simulink model "DrivePurePursuitSquat"  (R2025b)
settings: Solver=VariableStepAuto  StartTime=0.0  StopTime=120  RelTol=0.01  AbsTol=0.01  EnableMultiTasking=on
undefined symbols (not defined in the file): waypoints, X, Y, Z
libraries: sm_lib x71, nesl_utility x45, slpidlib x2, robotalgslib x1, sharedtransform x1
(part 4 of 4)

== system DrivePurePursuitSquat/Subsystem5 ==
  In2 : Inport
  wR_cmd : Inport  Port=2
  PID Controller : slpidlib/PID Controller  Controller=PID  Form=Parallel  TimeDomain=Continuous-time  UseExternalTs=off  SampleTime=-1  IntegratorMethod=Forward Euler  FilterMethod=Forward Euler  ControllerParametersSource=internal  P=5  I=0  UseKiTs=off  D=0  UseExternalDerivativeSource=off  N=100  UseFilter=on  TunerSelectOption=Transfer Function Based (PID Tuner App)  InitialConditionSource=internal  InitialConditionForIntegrator=0  InitialConditionForFilter=0  DifferentiatorICPrevScaledInput=0  ExternalReset=none  TrackingMode=off  Kt=1  LimitOutput=off  SatLimitsSource=internal  UpperSaturationLimit=inf  LowerSaturationLimit=-inf  LinearizeAsGain=on  AntiWindupMode=none  Kb=1  LimitIntegrator=off  UpperIntegratorSaturationLimit=inf  LowerIntegratorSaturationLimit=-inf  POutMin=[]  POutMax=[]  IOutMin=[]  IOutMax=[]  DOutMin=[]  DOutMax=[]  NOutMin=[]  NOutMax=[]  SumOutMin=[]  SumOutMax=[]  SaturationOutMin=[]  SaturationOutMax=[]  PParamMin=[]  PParamMax=[]  IParamMin=[]  IParamMax=[]  DParamMin=[]  DParamMax=[]  NParamMin=[]  NParamMax=[]  KbParamMin=[]  KbParamMax=[]  KtParamMin=[]  KtParamMax=[]  KbOutMin=[]  KbOutMax=[]  KtOutMin=[]  KtOutMax=[]  IntegratorOutMin=[]  IntegratorOutMax=[]  FilterOutMin=[]  FilterOutMax=[]  SumI1OutMin=[]  SumI1OutMax=[]  SumI2OutMin=[]  SumI2OutMax=[]  SumI3OutMin=[]  SumI3OutMax=[]  SumI4OutMin=[]  SumI4OutMax=[]  SumDOutMin=[]  SumDOutMax=[]  DifferentiatorOutMin=[]  DifferentiatorOutMax=[]  FilterDiffOutCoefMin=[]  FilterDiffOutCoefMax=[]  ReciprocalOutMin=[]  ReciprocalOutMax=[]  SumDenOutMin=[]  SumDenOutMax=[]  SumNumOutMin=[]  SumNumOutMax=[]  DivideOutMin=[]  DivideOutMax=[]  UdiffTsProdOutMin=[]  UdiffTsProdOutMax=[]  NTsProdOutMin=[]  NTsProdOutMax=[]  UintegralTsProdOutMin=[]  UintegralTsProdOutMax=[]  UngainTsProdOutMin=[]  UngainTsProdOutMax=[]  ClampingZeroOutDataTypeStr=Inherit: Inherit via back propagation  ClampingZeroOutMin=[]  ClampingZeroOutMax=[]  FilterDenConstantOutDataTypeStr=Inherit: Inherit via back propagation  FilterDenConstantOutMin=[]  FilterDenConstantOutMax=[]  PCopyOutDataTypeStr=Inherit: Inherit via back propagation  PCopyOutMin=[]  PCopyOutMax=[]  NCopyOutDataTypeStr=Inherit: Inherit via back propagation  NCopyOutMin=[]  NCopyOutMax=[]  IntegratorContinuousStateAttributes=''  IntegratorStateMustResolveToSignalObject=off  IntegratorRTWStateStorageClass=Auto  FilterContinuousStateAttributes=''  FilterStateMustResolveToSignalObject=off  FilterRTWStateStorageClass=Auto  ParallelPVariant=InternalParameters  IdealPVariant=Disabled  IVariant=InternalParameters  DVariant=InternalParameters  IntegratorVariant=Continuous  SatVariant=Disabled  AWVariant=Passthrough  PCopyVariant=Disabled  TRVariant=Disabled  FdbkBlocksVariant=Forward  IdealPFdbkVariant=Disabled  SatFdbkVariant=Disabled  DerivativeFilterVariant=ContFilter  NVariant=InternalParameters  NCopyVariant=Disabled  FilterICVariant=InternalICsFilter  IntegratorICVariant=InternalICs  ExternalResetVariant=Disabled  TRSumVariant=Passthrough  SumFdbkVariant=Disabled  SumVariant=Sum_PID  TsampFilterVariant=InternalTs  TsampNgainVariant=Passthrough  TsampIntegralVariant=Disabled_SignalSpec  ExternalSaturationOutDataTypeStr=Inherit: Same as second input  DerivativeSourceVariant=ErrorSignal  PreIntVariant=InternalPreInt
  Saturation : Saturate  UpperLimit=5  LowerLimit=-5
  Subtract : Sum  Inputs=+-
  Out1 : Outport
  wires:
  In2/1 -> Subtract/2
  Subtract/1 -> PID Controller/1
  Saturation/1 -> Out1/1
  PID Controller/1 -> Saturation/1
  wR_cmd/1 -> Subtract/1

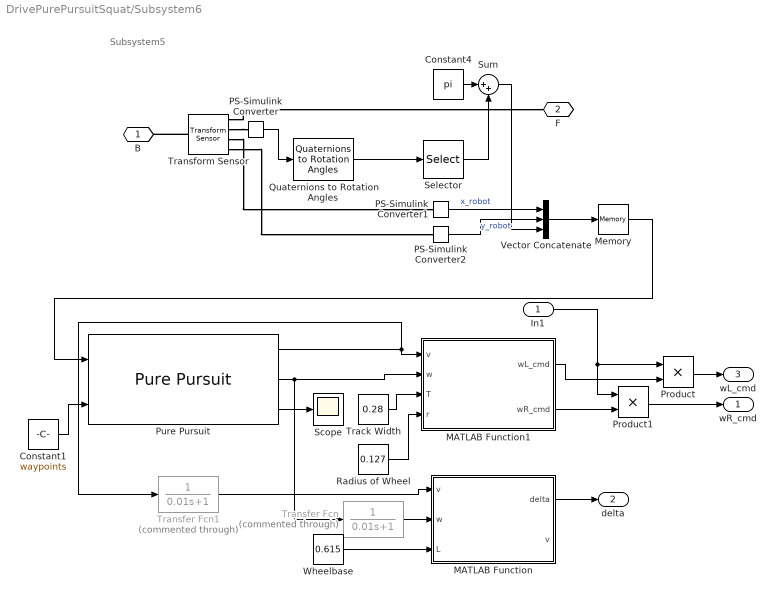
== system DrivePurePursuitSquat/Subsystem6 ==
  note: Subsystem5
  In1 : Inport
  Constant1 : Constant  Value=waypoints
  Constant4 : Constant  Value=pi
  MATLAB Function : MATLAB Function  TreatAsAtomicUnit=on
  MATLAB Function1 : MATLAB Function  TreatAsAtomicUnit=on
  Memory : Memory
  PS-Simulink Converter : nesl_utility/PS-Simulink Converter  PhysicalDomain=network_engine_domain  SubClassName=ps_output  LeftPortType=input  RightPortType=output  PseudoPeriodic=off  Frequencies=[]  VectorFormat=inherit  Unit=inherit  AffineConversion=off
  PS-Simulink Converter1 : nesl_utility/PS-Simulink Converter  PhysicalDomain=network_engine_domain  SubClassName=ps_output  LeftPortType=input  RightPortType=output  PseudoPeriodic=off  Frequencies=[]  VectorFormat=inherit  Unit=inherit  AffineConversion=off
  PS-Simulink Converter2 : nesl_utility/PS-Simulink Converter  PhysicalDomain=network_engine_domain  SubClassName=ps_output  LeftPortType=input  RightPortType=output  PseudoPeriodic=off  Frequencies=[]  VectorFormat=inherit  Unit=inherit  AffineConversion=off
  Product : Product
  Product1 : Product
  Pure Pursuit : robotalgslib/Pure Pursuit  DesiredLinearVelocityPort=off  DesiredLinearVelocity=0.7  MaxAngularVelocity=0.8  LookaheadDistancePort=off  LookaheadDistance=0.6  TargetDirPort=on  SimulateUsing=Code generation
      settings: LibrarySourceBlock=navlib/Control Algorithms/Pure Pursuit
  Quaternions to Rotation Angles : sharedtransform/Quaternions to Rotation Angles  rotationOrder=ZYX  aMode=aMode
  Radius of Wheel : Constant  Value=0.127
  Scope : Scope
      settings: ActiveDisplayYMinimum=-49.938512022124293  ActiveDisplayYMaximum=229.50278461957694
  Selector : Selector  InputPortWidth=3  IndexOptions=Index vector (dialog)  Indices=[1]  OutputSizes=1
  Sum : Sum  Inputs=|++
  Track Width : Constant  Value=0.28
  Transfer Fcn : TransferFcn  Commented=through  Denominator=[0.01 1]
  Transfer Fcn1 : TransferFcn  Commented=through  Denominator=[0.01 1]
  Transform Sensor : sm_lib/Frames and Transforms/Transform Sensor  MeasurementFrame=World  RotationSequence=XYX  SenseAngle=off  SenseAxis=off  SenseQ=on  SenseR=off  SenseRotationSequence=off  SenseOmegaX=off  SenseOmegaY=off  SenseOmegaZ=off  SenseOmega=off  SenseQDot=off  SenseRDot=off  SenseRotationSequenceDot=off  SenseAlphaX=off  SenseAlphaY=off  SenseAlphaZ=off  SenseAlpha=off  SenseQDDot=off  SenseRDDot=off  SenseX=on  SenseY=on  SenseZ=off  SenseXYZ=off  SenseRad=off  SenseAzim=off  SenseDist=off  SenseInc=off  SenseXDot=off  SenseYDot=off  SenseZDot=off  SenseXYZDot=off  SenseRadDot=off  SenseAzimDot=off  SenseDistDot=off  SenseIncDot=off  SenseXDDot=off  SenseYDDot=off  SenseZDDot=off  SenseXYZDDot=off  SenseRadDDot=off  SenseAzimDDot=off  SenseDistDDot=off  SenseIncDDot=off
  Vector Concatenate : Concatenate  NumInputs=3
  Wheelbase : Constant  Value=0.615
  B : PMIOPort  Side=Left
  F : PMIOPort  Port=2  Side=Right
  wR_cmd : Outport
  delta : Outport  Port=2
  wL_cmd : Outport  Port=3
  wires:
  Pure Pursuit/2 -> MATLAB Function1/2(w), Transfer Fcn/1
  Transfer Fcn1/1 -> MATLAB Function/1("v ")
  Transfer Fcn/1 -> MATLAB Function/2(w)
  Constant1/1 -> Pure Pursuit/2
  Radius of Wheel/1 -> MATLAB Function1/4(r)
  Track Width/1 -> MATLAB Function1/3(T)
  Wheelbase/1 -> MATLAB Function/3(L)
  Pure Pursuit/1 -> MATLAB Function1/1(v), Transfer Fcn1/1
  Pure Pursuit/3 -> Scope/1
  Memory/1 -> Pure Pursuit/1
  In1/1 -> Product/1, Product1/1
  MATLAB Function1/1(wL_cmd) -> Product/2
  Product/1 -> wL_cmd/1
  MATLAB Function1/2(wR_cmd) -> Product1/2
  Product1/1 -> wR_cmd/1
  MATLAB Function/1(delta) -> delta/1
  Sum/1 -> Vector Concatenate/3
  Selector/1 -> Sum/2
  Constant4/1 -> Sum/1
  PS-Simulink Converter2/1 -> Vector Concatenate/2  "y_robot"
  PS-Simulink Converter1/1 -> Vector Concatenate/1  "x_robot"
  Vector Concatenate/1 -> Memory/1
  PS-Simulink Converter/1 -> Quaternions to Rotation Angles/1
  Quaternions to Rotation Angles/1 -> Selector/1
  connections:
  Transform Sensor/RConn1 -- F/RConn1
  Transform Sensor/LConn1 -- B/RConn1
  Transform Sensor/RConn3 -- PS-Simulink Converter1/LConn1
  Transform Sensor/RConn2 -- PS-Simulink Converter/LConn1
  Transform Sensor/RConn4 -- PS-Simulink Converter2/LConn1

== system DrivePurePursuitSquat/Subsystem7 ==
  wL_cmd : Inport
  In2 : Inport  Port=2
  PID Controller : slpidlib/PID Controller  Controller=PID  Form=Parallel  TimeDomain=Continuous-time  UseExternalTs=off  SampleTime=-1  IntegratorMethod=Forward Euler  FilterMethod=Forward Euler  ControllerParametersSource=internal  P=5  I=0  UseKiTs=off  D=0  UseExternalDerivativeSource=off  N=100  UseFilter=on  TunerSelectOption=Transfer Function Based (PID Tuner App)  InitialConditionSource=internal  InitialConditionForIntegrator=0  InitialConditionForFilter=0  DifferentiatorICPrevScaledInput=0  ExternalReset=none  TrackingMode=off  Kt=1  LimitOutput=off  SatLimitsSource=internal  UpperSaturationLimit=inf  LowerSaturationLimit=-inf  LinearizeAsGain=on  AntiWindupMode=none  Kb=1  LimitIntegrator=off  UpperIntegratorSaturationLimit=inf  LowerIntegratorSaturationLimit=-inf  POutMin=[]  POutMax=[]  IOutMin=[]  IOutMax=[]  DOutMin=[]  DOutMax=[]  NOutMin=[]  NOutMax=[]  SumOutMin=[]  SumOutMax=[]  SaturationOutMin=[]  SaturationOutMax=[]  PParamMin=[]  PParamMax=[]  IParamMin=[]  IParamMax=[]  DParamMin=[]  DParamMax=[]  NParamMin=[]  NParamMax=[]  KbParamMin=[]  KbParamMax=[]  KtParamMin=[]  KtParamMax=[]  KbOutMin=[]  KbOutMax=[]  KtOutMin=[]  KtOutMax=[]  IntegratorOutMin=[]  IntegratorOutMax=[]  FilterOutMin=[]  FilterOutMax=[]  SumI1OutMin=[]  SumI1OutMax=[]  SumI2OutMin=[]  SumI2OutMax=[]  SumI3OutMin=[]  SumI3OutMax=[]  SumI4OutMin=[]  SumI4OutMax=[]  SumDOutMin=[]  SumDOutMax=[]  DifferentiatorOutMin=[]  DifferentiatorOutMax=[]  FilterDiffOutCoefMin=[]  FilterDiffOutCoefMax=[]  ReciprocalOutMin=[]  ReciprocalOutMax=[]  SumDenOutMin=[]  SumDenOutMax=[]  SumNumOutMin=[]  SumNumOutMax=[]  DivideOutMin=[]  DivideOutMax=[]  UdiffTsProdOutMin=[]  UdiffTsProdOutMax=[]  NTsProdOutMin=[]  NTsProdOutMax=[]  UintegralTsProdOutMin=[]  UintegralTsProdOutMax=[]  UngainTsProdOutMin=[]  UngainTsProdOutMax=[]  ClampingZeroOutDataTypeStr=Inherit: Inherit via back propagation  ClampingZeroOutMin=[]  ClampingZeroOutMax=[]  FilterDenConstantOutDataTypeStr=Inherit: Inherit via back propagation  FilterDenConstantOutMin=[]  FilterDenConstantOutMax=[]  PCopyOutDataTypeStr=Inherit: Inherit via back propagation  PCopyOutMin=[]  PCopyOutMax=[]  NCopyOutDataTypeStr=Inherit: Inherit via back propagation  NCopyOutMin=[]  NCopyOutMax=[]  IntegratorContinuousStateAttributes=''  IntegratorStateMustResolveToSignalObject=off  IntegratorRTWStateStorageClass=Auto  FilterContinuousStateAttributes=''  FilterStateMustResolveToSignalObject=off  FilterRTWStateStorageClass=Auto  ParallelPVariant=InternalParameters  IdealPVariant=Disabled  IVariant=InternalParameters  DVariant=InternalParameters  IntegratorVariant=Continuous  SatVariant=Disabled  AWVariant=Passthrough  PCopyVariant=Disabled  TRVariant=Disabled  FdbkBlocksVariant=Forward  IdealPFdbkVariant=Disabled  SatFdbkVariant=Disabled  DerivativeFilterVariant=ContFilter  NVariant=InternalParameters  NCopyVariant=Disabled  FilterICVariant=InternalICsFilter  IntegratorICVariant=InternalICs  ExternalResetVariant=Disabled  TRSumVariant=Passthrough  SumFdbkVariant=Disabled  SumVariant=Sum_PID  TsampFilterVariant=InternalTs  TsampNgainVariant=Passthrough  TsampIntegralVariant=Disabled_SignalSpec  ExternalSaturationOutDataTypeStr=Inherit: Same as second input  DerivativeSourceVariant=ErrorSignal  PreIntVariant=InternalPreInt
  Saturation : Saturate  UpperLimit=5  LowerLimit=-5
  Subtract : Sum  Inputs=+-
  Out1 : Outport
  wires:
  In2/1 -> Subtract/2
  Subtract/1 -> PID Controller/1
  Saturation/1 -> Out1/1
  PID Controller/1 -> Saturation/1
  wL_cmd/1 -> Subtract/1

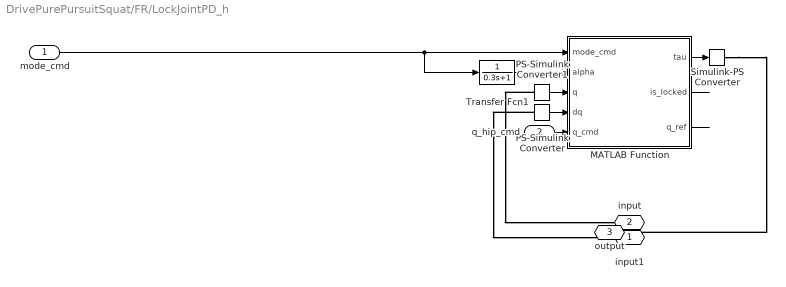
== system DrivePurePursuitSquat/FR/LockJointPD_h ==
  mode_cmd : Inport
  q_hip_cmd : Inport  Port=2
  MATLAB Function : MATLAB Function  TreatAsAtomicUnit=on  SystemSampleTime=0.002
  PS-Simulink Converter : nesl_utility/PS-Simulink Converter  PhysicalDomain=network_engine_domain  SubClassName=ps_output  LeftPortType=input  RightPortType=output  PseudoPeriodic=off  Frequencies=[]  VectorFormat=inherit  Unit=inherit  AffineConversion=off
  PS-Simulink Converter1 : nesl_utility/PS-Simulink Converter  PhysicalDomain=network_engine_domain  SubClassName=ps_output  LeftPortType=input  RightPortType=output  PseudoPeriodic=off  Frequencies=[]  VectorFormat=inherit  Unit=inherit  AffineConversion=off
  Simulink-PS Converter : nesl_utility/Simulink-PS Converter  PhysicalDomain=network_engine_domain  SubClassName=ps_input  LeftPortType=input  RightPortType=output  PseudoPeriodic=off  Frequencies=[]  NoiseDistribution=none  NoiseParameters=[]  Unit=1  AffineConversion=off  FilteringAndDerivatives=provide  SimscapeFilterOrder=1  InputFilterTimeConstant=0.001  UdotUserProvided=0
  Transfer Fcn1 : TransferFcn  Denominator=[0.3 1]
  input1 : PMIOPort  Side=Left
  input : PMIOPort  Port=2  Side=Left
  output : PMIOPort  Port=3  Side=Right
  wires:
  PS-Simulink Converter1/1 -> MATLAB Function/3(q)
  q_hip_cmd/1 -> MATLAB Function/5(q_cmd)
  MATLAB Function/2(is_locked) -> ?
  MATLAB Function/1(tau) -> Simulink-PS Converter/1
  PS-Simulink Converter/1 -> MATLAB Function/4(dq)
  mode_cmd/1 -> Transfer Fcn1/1, MATLAB Function/1(mode_cmd)
  Transfer Fcn1/1 -> MATLAB Function/2(alpha)
  MATLAB Function/3(q_ref) -> ?
  connections:
  PS-Simulink Converter1/LConn1 -- input/RConn1
  PS-Simulink Converter/LConn1 -- input1/RConn1
  Simulink-PS Converter/RConn1 -- output/RConn1

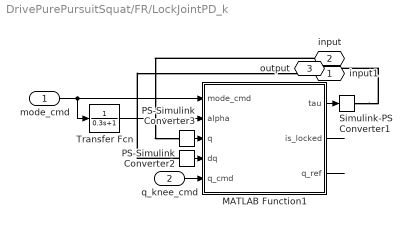
== system DrivePurePursuitSquat/FR/LockJointPD_k ==
  mode_cmd : Inport
  q_knee_cmd : Inport  Port=2
  MATLAB Function1 : MATLAB Function  TreatAsAtomicUnit=on  SystemSampleTime=0.002
  PS-Simulink Converter2 : nesl_utility/PS-Simulink Converter  PhysicalDomain=network_engine_domain  SubClassName=ps_output  LeftPortType=input  RightPortType=output  PseudoPeriodic=off  Frequencies=[]  VectorFormat=inherit  Unit=inherit  AffineConversion=off
  PS-Simulink Converter3 : nesl_utility/PS-Simulink Converter  PhysicalDomain=network_engine_domain  SubClassName=ps_output  LeftPortType=input  RightPortType=output  PseudoPeriodic=off  Frequencies=[]  VectorFormat=inherit  Unit=inherit  AffineConversion=off
  Simulink-PS Converter1 : nesl_utility/Simulink-PS Converter  PhysicalDomain=network_engine_domain  SubClassName=ps_input  LeftPortType=input  RightPortType=output  PseudoPeriodic=off  Frequencies=[]  NoiseDistribution=none  NoiseParameters=[]  Unit=1  AffineConversion=off  FilteringAndDerivatives=provide  SimscapeFilterOrder=1  InputFilterTimeConstant=0.001  UdotUserProvided=0
  Transfer Fcn : TransferFcn  Denominator=[0.3 1]
  input1 : PMIOPort  Side=Left
  input : PMIOPort  Port=2  Side=Left
  output : PMIOPort  Port=3  Side=Right
  wires:
  q_knee_cmd/1 -> MATLAB Function1/5(q_cmd)
  Transfer Fcn/1 -> MATLAB Function1/2(alpha)
  PS-Simulink Converter3/1 -> MATLAB Function1/3(q)
  PS-Simulink Converter2/1 -> MATLAB Function1/4(dq)
  mode_cmd/1 -> Transfer Fcn/1, MATLAB Function1/1(mode_cmd)
  MATLAB Function1/1(tau) -> Simulink-PS Converter1/1
  MATLAB Function1/3(q_ref) -> ?
  MATLAB Function1/2(is_locked) -> ?
  connections:
  input/RConn1 -- PS-Simulink Converter3/LConn1
  PS-Simulink Converter2/LConn1 -- input1/RConn1
  Simulink-PS Converter1/RConn1 -- output/RConn1

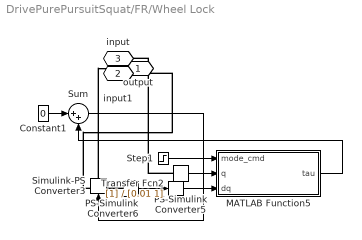
== system DrivePurePursuitSquat/FR/Wheel Lock ==
  Constant1 : Constant  Value=0
  MATLAB Function5 : MATLAB Function  TreatAsAtomicUnit=on
  PS-Simulink Converter5 : nesl_utility/PS-Simulink Converter  PhysicalDomain=network_engine_domain  SubClassName=ps_output  LeftPortType=input  RightPortType=output  PseudoPeriodic=off  Frequencies=[]  VectorFormat=inherit  Unit=inherit  AffineConversion=off
  PS-Simulink Converter6 : nesl_utility/PS-Simulink Converter  PhysicalDomain=network_engine_domain  SubClassName=ps_output  LeftPortType=input  RightPortType=output  PseudoPeriodic=off  Frequencies=[]  VectorFormat=inherit  Unit=inherit  AffineConversion=off
  Simulink-PS Converter3 : nesl_utility/Simulink-PS Converter  PhysicalDomain=network_engine_domain  SubClassName=ps_input  LeftPortType=input  RightPortType=output  PseudoPeriodic=off  Frequencies=[]  NoiseDistribution=none  NoiseParameters=[]  Unit=1  AffineConversion=off  FilteringAndDerivatives=filter  SimscapeFilterOrder=2  InputFilterTimeConstant=0.01  UdotUserProvided=0
  Step1 : Step  Time=1000  Before=1  After=0  SampleTime=0
  Sum : Sum  Inputs=|++
  Transfer Fcn2 : TransferFcn  Denominator=[0.01 1]
  output : PMIOPort  Side=Left
  input1 : PMIOPort  Port=2  Side=Right
  input : PMIOPort  Port=3  Side=Right
  wires:
  Transfer Fcn2/1 -> MATLAB Function5/3(dq)
  PS-Simulink Converter5/1 -> MATLAB Function5/2(q)
  MATLAB Function5/1(tau) -> Sum/2
  Step1/1 -> MATLAB Function5/1(mode_cmd)
  Constant1/1 -> Sum/1
  Sum/1 -> Simulink-PS Converter3/1
  PS-Simulink Converter6/1 -> Transfer Fcn2/1
  connections:
  PS-Simulink Converter6/LConn1 -- input1/RConn1
  Simulink-PS Converter3/RConn1 -- output/RConn1
  PS-Simulink Converter5/LConn1 -- input/RConn1

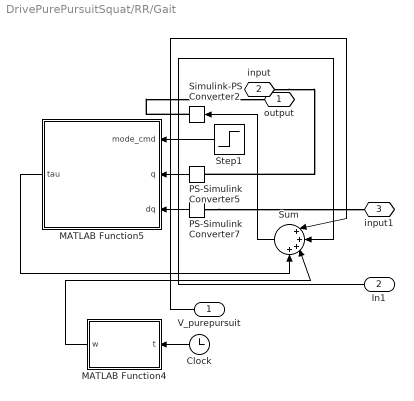
== system DrivePurePursuitSquat/RR/Gait ==
  V_purepursuit : Inport
  In1 : Inport  Port=2
  Clock : Clock
  MATLAB Function4 : MATLAB Function  TreatAsAtomicUnit=on
  MATLAB Function5 : MATLAB Function  TreatAsAtomicUnit=on
  PS-Simulink Converter5 : nesl_utility/PS-Simulink Converter  PhysicalDomain=network_engine_domain  SubClassName=ps_output  LeftPortType=input  RightPortType=output  PseudoPeriodic=off  Frequencies=[]  VectorFormat=inherit  Unit=inherit  AffineConversion=off
  PS-Simulink Converter7 : nesl_utility/PS-Simulink Converter  PhysicalDomain=network_engine_domain  SubClassName=ps_output  LeftPortType=input  RightPortType=output  PseudoPeriodic=off  Frequencies=[]  VectorFormat=inherit  Unit=inherit  AffineConversion=off
  Simulink-PS Converter2 : nesl_utility/Simulink-PS Converter  PhysicalDomain=network_engine_domain  SubClassName=ps_input  LeftPortType=input  RightPortType=output  PseudoPeriodic=off  Frequencies=[]  NoiseDistribution=none  NoiseParameters=[]  Unit=1  AffineConversion=off  FilteringAndDerivatives=provide  SimscapeFilterOrder=1  InputFilterTimeConstant=0.001  UdotUserProvided=0
  Step1 : Step  Time=135  Before=1  After=0  SampleTime=0
  Sum : Sum  Inputs=|++++
  output : PMIOPort  Side=Left
  input : PMIOPort  Port=2  Side=Right
  input1 : PMIOPort  Port=3  Side=Right
  wires:
  MATLAB Function4/1(w) -> Sum/3
  PS-Simulink Converter5/1 -> MATLAB Function5/2(q)
  MATLAB Function5/1(tau) -> Sum/4
  V_purepursuit/1 -> Sum/1
  Clock/1 -> MATLAB Function4/1(t)
  Step1/1 -> MATLAB Function5/1(mode_cmd)
  Sum/1 -> Simulink-PS Converter2/1
  PS-Simulink Converter7/1 -> MATLAB Function5/3(dq)
  In1/1 -> Sum/2
  connections:
  Simulink-PS Converter2/RConn1 -- output/RConn1
  input/RConn1 -- PS-Simulink Converter5/LConn1
  PS-Simulink Converter7/LConn1 -- input1/RConn1

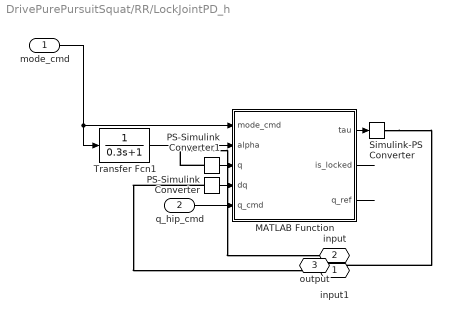
== system DrivePurePursuitSquat/RR/LockJointPD_h ==
  mode_cmd : Inport
  q_hip_cmd : Inport  Port=2
  MATLAB Function : MATLAB Function  TreatAsAtomicUnit=on  SystemSampleTime=0.002
  PS-Simulink Converter : nesl_utility/PS-Simulink Converter  PhysicalDomain=network_engine_domain  SubClassName=ps_output  LeftPortType=input  RightPortType=output  PseudoPeriodic=off  Frequencies=[]  VectorFormat=inherit  Unit=inherit  AffineConversion=off
  PS-Simulink Converter1 : nesl_utility/PS-Simulink Converter  PhysicalDomain=network_engine_domain  SubClassName=ps_output  LeftPortType=input  RightPortType=output  PseudoPeriodic=off  Frequencies=[]  VectorFormat=inherit  Unit=inherit  AffineConversion=off
  Simulink-PS Converter : nesl_utility/Simulink-PS Converter  PhysicalDomain=network_engine_domain  SubClassName=ps_input  LeftPortType=input  RightPortType=output  PseudoPeriodic=off  Frequencies=[]  NoiseDistribution=none  NoiseParameters=[]  Unit=1  AffineConversion=off  FilteringAndDerivatives=provide  SimscapeFilterOrder=1  InputFilterTimeConstant=0.001  UdotUserProvided=0
  Transfer Fcn1 : TransferFcn  Denominator=[0.3 1]
  input1 : PMIOPort  Side=Left
  input : PMIOPort  Port=2  Side=Left
  output : PMIOPort  Port=3  Side=Right
  wires:
  PS-Simulink Converter1/1 -> MATLAB Function/3(q)
  mode_cmd/1 -> Transfer Fcn1/1, MATLAB Function/1(mode_cmd)
  Transfer Fcn1/1 -> MATLAB Function/2(alpha)
  q_hip_cmd/1 -> MATLAB Function/5(q_cmd)
  PS-Simulink Converter/1 -> MATLAB Function/4(dq)
  MATLAB Function/1(tau) -> Simulink-PS Converter/1
  MATLAB Function/3(q_ref) -> ?
  MATLAB Function/2(is_locked) -> ?
  connections:
  PS-Simulink Converter1/LConn1 -- input/RConn1
  PS-Simulink Converter/LConn1 -- input1/RConn1
  Simulink-PS Converter/RConn1 -- output/RConn1

== system DrivePurePursuitSquat/RR/LockJointPD_k ==
  mode_cmd : Inport
  q_knee_cmd : Inport  Port=2
  MATLAB Function1 : MATLAB Function  TreatAsAtomicUnit=on  SystemSampleTime=0.002
  PS-Simulink Converter2 : nesl_utility/PS-Simulink Converter  PhysicalDomain=network_engine_domain  SubClassName=ps_output  LeftPortType=input  RightPortType=output  PseudoPeriodic=off  Frequencies=[]  VectorFormat=inherit  Unit=inherit  AffineConversion=off
  PS-Simulink Converter3 : nesl_utility/PS-Simulink Converter  PhysicalDomain=network_engine_domain  SubClassName=ps_output  LeftPortType=input  RightPortType=output  PseudoPeriodic=off  Frequencies=[]  VectorFormat=inherit  Unit=inherit  AffineConversion=off
  Simulink-PS Converter1 : nesl_utility/Simulink-PS Converter  PhysicalDomain=network_engine_domain  SubClassName=ps_input  LeftPortType=input  RightPortType=output  PseudoPeriodic=off  Frequencies=[]  NoiseDistribution=none  NoiseParameters=[]  Unit=1  AffineConversion=off  FilteringAndDerivatives=provide  SimscapeFilterOrder=1  InputFilterTimeConstant=0.001  UdotUserProvided=0
  Transfer Fcn : TransferFcn  Denominator=[0.3 1]
  input1 : PMIOPort  Side=Left
  input : PMIOPort  Port=2  Side=Left
  output : PMIOPort  Port=3  Side=Right
  wires:
  PS-Simulink Converter2/1 -> MATLAB Function1/4(dq)
  mode_cmd/1 -> Transfer Fcn/1, MATLAB Function1/1(mode_cmd)
  Transfer Fcn/1 -> MATLAB Function1/2(alpha)
  q_knee_cmd/1 -> MATLAB Function1/5(q_cmd)
  PS-Simulink Converter3/1 -> MATLAB Function1/3(q)
  MATLAB Function1/1(tau) -> Simulink-PS Converter1/1
  MATLAB Function1/2(is_locked) -> ?
  MATLAB Function1/3(q_ref) -> ?
  connections:
  input/RConn1 -- PS-Simulink Converter3/LConn1
  Simulink-PS Converter1/RConn1 -- output/RConn1
  PS-Simulink Converter2/LConn1 -- input1/RConn1

== matlab function DrivePurePursuitSquat/RL/MATLAB Function1 ==
  data: mode_cmd input; alpha input; tau output; q input; dq input; q_cmd input; is_locked output; q_ref output
function [tau, is_locked, q_ref] = LockJointPD(mode_cmd, alpha, q, dq, q_cmd)
%#codegen
% mode_cmd: 0=Walk (track q_cmd), 1=Wheeled (lock current angle)
% alpha   : [0,1] smoothing factor (TransferFcn output), 0=fully walking, 1=fully locked
% q,dq    : joint angle/angular velocity
% q_cmd   : walk/stand target angle (radians)
Kp = 1200.0;   % Starting value, tune per joint
Kd =   20.0;
tau_lim = 300.0;
m = uint8(mode_cmd ~= 0);     % Standardize to uint8(0/1)
a = double(alpha);
persistent q_hold last_mode
if isempty(q_hold),    q_hold    = q;        end   % double
if isempty(last_mode), last_mode = uint8(0); end   % uint8
% Rising edge: 0->1, latch current angle
if (last_mode == uint8(0)) && (m ~= uint8(0))
    q_hold = q;
end
last_mode = m;
% Reference angle: interpolate between "hold angle" and "target angle"
q_ref  = a*q_hold + (1-a)*q_cmd;
dq_ref = 0.0;
% PD
tau = Kp*(q_ref - q) + Kd*(dq_ref - dq);
% Saturation
tau = max(min(tau, tau_lim), -tau_lim);
% Debug flag: is leg lock dominant
is_locked = (a > 0.5);     % Can also output m==1
end

== matlab function DrivePurePursuitSquat/Subsystem6/MATLAB Function1 ==
  data: v input; wL_cmd output; w input; T input; r input; wR_cmd output
function [wL_cmd, wR_cmd] = wheelSpeedCmd(v, w, T, r)

vL = v - 0.5*T*w;
vR = v + 0.5*T*w;

wL_cmd = vL / r;
wR_cmd = vR / r;
end

== matlab function DrivePurePursuitSquat/Subsystem6/MATLAB Function ==
  data: v input; delta output; w input; L input; v output
function [delta, v] = Diff2Ackermann(v, w, L)
% input: 
%   v - Linear velocity (m/s)
%   w - Angular velocity (rad/s)
%   L - Wheelbase (m)
%
% output:
%   delta - front wheel rotation angel (rad)
%   v     -  velocity(m/s)
if abs(v) < 1e-3
    delta = 0;
else
    delta = atan(L * w / v);   % pure pursuit function
end

== matlab function DrivePurePursuitSquat/RL/MATLAB Function2 ==
  data: t input; w output
function w = wheel_speed(t)


Tsw  = 105;  
Tacc = 2;     
V    = 100;   
Tdec_start = 125;   
Tdec = 3;           

if t < Tsw
    w = 0;


elseif t < Tsw + Tacc
    u = (t - Tsw) / Tacc;
    w = u * V;


elseif t < Tdec_start
    w = V;


elseif t < Tdec_start + Tdec
    u = (t - Tdec_start) / Tdec;  
    w = V * (1 - u);

else
    w = 0;
end
end

== matlab function DrivePurePursuitSquat/RL/MATLAB Function3 ==
  data: brake_en input; tau output; w input
function tau = BrakeTorque(brake_en, w)


Kb = 30.0;       
tau_max = 150.0; 
w_eps = 0.05;    

if brake_en == 0
    tau = 0.0;   
    return;
end

if abs(w) < w_eps
    tau = 0.0;
else
   
    tau = -Kb * w;
end

if tau >  tau_max, tau =  tau_max; end
if tau < -tau_max, tau = -tau_max; end
end

== matlab function DrivePurePursuitSquat/FL_climb/MATLAB Function2 ==
  data: t input; q output; mode_cmd input
function q = hip_FL_motion(t, mode_cmd)


T_squat_start = 102;
T_climb_start = 130;


if (mode_cmd == 1) || (t < T_squat_start); q = 0; return; end

if t < T_climb_start
    tau = t - T_squat_start;
    q_stand = 0; q_squat = deg2rad(35);
    T1 = 3; T2 = 15; T3 = 3;
    if tau < T1; u=tau/T1; q=(1-u)*q_stand+u*q_squat;
    elseif tau < T1+T2; q=q_squat;
    elseif tau < T1+T2+T3; u=(tau-(T1+T2))/T3; q=(1-u)*q_squat+u*q_stand;
    else; q=q_stand; end
    return;
end

tau = t - T_climb_start;


    q_neutral = 0;
    q_fwd     = deg2rad(-5); 
    
   
    if tau < 2.0
        u = tau / 2.0;
        q = (1-u)*q_neutral + u*q_fwd;
        
    elseif tau < 4.0
        q = q_fwd;
        
    elseif tau < 8.0
        dt = tau - 4.0;
        u = dt / 4.0;
        u_smooth = 0.5 * (1 - cos(u * pi));
        q = (1-u_smooth)*q_fwd + u_smooth*q_neutral;
        
    else
        q = q_neutral;
    end
end

== matlab function DrivePurePursuitSquat/FL_climb/MATLAB Function3 ==
  data: t input; q output; mode_cmd input
function q = knee_FL_motion(t, mode_cmd)

T_squat_start = 102;
T_climb_start = 130;

if (mode_cmd == 1) || (t < T_squat_start); q = 0; return; end
if t < T_climb_start
    tau = t - T_squat_start;
    q_stand = 0; q_squat = -deg2rad(70);
    T1 = 3; T2 = 15; T3 = 3;
    if tau < T1; u=tau/T1; q=(1-u)*q_stand+u*q_squat;
    elseif tau < T1+T2; q=q_squat;
    elseif tau < T1+T2+T3; u=(tau-(T1+T2))/T3; q=(1-u)*q_squat+u*q_stand;
    else; q=q_stand; end
    return;
end

 tau = t - T_climb_start;

q_stand = deg2rad(0);
    q_lift  = deg2rad(-20);
    
 
    if tau < 2.0
        u = tau / 2.0;
        lift_scale = sin(u * pi); 
        q = q_stand + lift_scale * (q_lift - q_stand);
        
  
    else
        q = q_stand;
    end
end

== matlab function DrivePurePursuitSquat/RR/LockJointPD_k/MATLAB Function1 ==
  data: mode_cmd input; alpha input; tau output; q input; dq input; q_cmd input; is_locked output; q_ref output
function [tau, is_locked, q_ref] = LockJointPD(mode_cmd, alpha, q, dq, q_cmd)
%#codegen
% mode_cmd: 0=Walk (track q_cmd), 1=Wheeled (lock current angle)
% alpha   : [0,1] smoothing factor (TransferFcn output), 0=fully walking, 1=fully locked
% q,dq    : joint angle/angular velocity
% q_cmd   : walk/stand target angle (radians)
Kp = 1200.0;   % Starting value, tune per joint
Kd =   20.0;
tau_lim = 300.0;
m = uint8(mode_cmd ~= 0);     % Standardize to uint8(0/1)
a = double(alpha);
persistent q_hold last_mode
if isempty(q_hold),    q_hold    = q;        end   % double
if isempty(last_mode), last_mode = uint8(0); end   % uint8
% Rising edge: 0->1, latch current angle
if (last_mode == uint8(0)) && (m ~= uint8(0))
    q_hold = q;
end
last_mode = m;
% Reference angle: interpolate between "hold angle" and "target angle"
q_ref  = a*q_hold + (1-a)*q_cmd;
dq_ref = 0.0;
% PD
tau = Kp*(q_ref - q) + Kd*(dq_ref - dq);
% Saturation
tau = max(min(tau, tau_lim), -tau_lim);
% Debug flag: is leg lock dominant
is_locked = (a > 0.5);     % Can also output m==1
end

== matlab function DrivePurePursuitSquat/RR/MATLAB Function3 ==
  data: brake_en input; tau output; w input
function tau = BrakeTorque(brake_en, w)


Kb = 30.0;       
tau_max = 150.0; 
w_eps = 0.05;    

if brake_en == 0
    tau = 0.0;   
    return;
end


if abs(w) < w_eps
    tau = 0.0;
else
    
    tau = -Kb * w;
end


if tau >  tau_max, tau =  tau_max; end
if tau < -tau_max, tau = -tau_max; end
end

== matlab function DrivePurePursuitSquat/FR_climb/MATLAB Function1 ==
  data: t input; q output; mode_cmd input
function q = hip_FR_motion(t, mode_cmd)


T_squat_start = 102;
T_climb_start = 130;


if (mode_cmd == 1) || (t < T_squat_start); q = 0; return; end
if t < T_climb_start
    tau = t - T_squat_start;
    q_stand = 0; q_squat = deg2rad(35);
    T1 = 3; T2 = 15; T3 = 3;
    if tau < T1; u=tau/T1; q=(1-u)*q_stand+u*q_squat;
    elseif tau < T1+T2; q=q_squat;
    elseif tau < T1+T2+T3; u=(tau-(T1+T2))/T3; q=(1-u)*q_squat+u*q_stand;
    else; q=q_stand; end
    return;
end


tau = t - T_climb_start;

q_neutral = 0;
    q_fwd     = deg2rad(-5);
    
  
    if tau < 4.0
        q = q_neutral;

  
    elseif tau < 8.0
        dt = tau - 4.0;
        u = dt / 4.0;
        q = (1-u)*q_neutral + u*q_fwd;
        

    elseif tau < 12.0
        dt = tau - 8.0;
        u = dt / 6.0;
        u_smooth = 0.5 * (1 - cos(u * pi));
        q = (1-u_smooth)*q_fwd + u_smooth*q_neutral;
        
    else
        q = q_neutral;
    end
end

== matlab function DrivePurePursuitSquat/FR_climb/MATLAB Function4 ==
  data: t input; q output; mode_cmd input
function q = knee_FR_motion(t, mode_cmd)


T_squat_start = 102;
T_climb_start = 130;


if (mode_cmd == 1) || (t < T_squat_start); q = 0; return; end
if t < T_climb_start
    tau = t - T_squat_start;
    q_stand = 0; q_squat = -deg2rad(70);
    T1 = 3; T2 = 15; T3 = 3;
    if tau < T1; u=tau/T1; q=(1-u)*q_stand+u*q_squat;
    elseif tau < T1+T2; q=q_squat;
    elseif tau < T1+T2+T3; u=(tau-(T1+T2))/T3; q=(1-u)*q_squat+u*q_stand;
    else; q=q_stand; end
    return;
end


tau = t - T_climb_start;

q_stand = deg2rad(0);
    q_lift  = deg2rad(-20);

    if tau < 4.0
        q = q_stand;
        

    elseif tau < 8.0
        dt = tau - 4.0;
        u = dt / 4.0;
        lift_scale = sin(u * pi);
        q = q_stand + lift_scale * (q_lift - q_stand);
        
    else
        q = q_stand;
    end
end

== matlab function DrivePurePursuitSquat/RL_climb/MATLAB Function2 ==
  data: t input; q output; mode_cmd input
function q = hip_RL_motion(t, mode_cmd)


T_squat_start = 102;
T_climb_start = 130; 

if (mode_cmd == 1) || (t < T_squat_start); q = 0; return; end

if t < T_climb_start
    tau = t - T_squat_start;
    q_stand = 0; q_squat = deg2rad(35);
    T1 = 3; T2 = 15; T3 = 3;
    if tau < T1; u=tau/T1; q=(1-u)*q_stand+u*q_squat;
    elseif tau < T1+T2; q=q_squat;
    elseif tau < T1+T2+T3; u=(tau-(T1+T2))/T3; q=(1-u)*q_squat+u*q_stand;
    else; q=q_stand;
    end
    return;
end

tau = t - T_climb_start;

q_neutral = 0;
    q_push    = deg2rad(15);
    

    if tau < 4.0
        q = q_neutral;
        
  
    elseif tau < 8.0
        dt = tau - 4.0;
        u = dt / 4.0;
        u_smooth = 0.5 * (1 - cos(u * pi));
        q = (1-u_smooth)*q_neutral + u_smooth*q_push;
        
   
    elseif tau < 10.0
        dt = tau - 8.0;
        u = dt / 2.0;
        q = (1-u)*q_push + u*q_neutral;
        
    else
        q = q_neutral;
    end
end

== matlab function DrivePurePursuitSquat/RL_climb/MATLAB Function3 ==
  data: t input; q output; mode_cmd input
function q = knee_RL_motion(t, mode_cmd)


T_squat_start = 102;
T_climb_start = 130;


if (mode_cmd == 1) || (t < T_squat_start); q = 0; return; end
if t < T_climb_start
    tau = t - T_squat_start;
    q_stand = 0; q_squat = -deg2rad(70);
    T1 = 3; T2 = 15; T3 = 3;
    if tau < T1; u=tau/T1; q=(1-u)*q_stand+u*q_squat;
    elseif tau < T1+T2; q=q_squat;
    elseif tau < T1+T2+T3; u=(tau-(T1+T2))/T3; q=(1-u)*q_squat+u*q_stand;
    else; q=q_stand;
    end
    return;
end


tau = t - T_climb_start;

q_stand = deg2rad(0);
    q_lift  = deg2rad(-20);
    
 
    if tau < 8.0
        q = q_stand;
        
   
    elseif tau < 10.0
        dt = tau - 8.0;
        u = dt / 2.0;
        lift_scale = sin(u * pi);
        q = q_stand + lift_scale * (q_lift - q_stand);
        
    else
        q = q_stand;
    end
end

== matlab function DrivePurePursuitSquat/RR_climb/MATLAB Function2 ==
  data: t input; q output; mode_cmd input
function q = hip_RR_motion(t, mode_cmd)

T_squat_start = 102;
T_climb_start = 130; 

if (mode_cmd == 1) || (t < T_squat_start); q = 0; return; end

if t < T_climb_start
    tau = t - T_squat_start;
    q_stand = 0; q_squat = deg2rad(35);
    T1 = 3; T2 = 15; T3 = 3;
    if tau < T1; u=tau/T1; q=(1-u)*q_stand+u*q_squat;
    elseif tau < T1+T2; q=q_squat;
    elseif tau < T1+T2+T3; u=(tau-(T1+T2))/T3; q=(1-u)*q_squat+u*q_stand;
    else; q=q_stand;
    end
    return;
end


tau = t - T_climb_start;

q_neutral = 0;
    q_push    = deg2rad(15);
    
    
    if tau < 4.0
        q = q_neutral;
        
  
    elseif tau < 8.0
        dt = tau - 4.0;
        u = dt / 4.0;
        u_smooth = 0.5 * (1 - cos(u * pi));
        q = (1-u_smooth)*q_neutral + u_smooth*q_push;
        
  
    elseif tau < 10.0
        q = q_push;

    
    elseif tau < 12.0
        dt = tau - 10.0;
        u = dt / 2.0;
        q = (1-u)*q_push + u*q_neutral;
        
    else
        q = q_neutral;
    end
end

== matlab function DrivePurePursuitSquat/RR_climb/MATLAB Function4 ==
  data: t input; q output; mode_cmd input
function q = knee_RR_motion(t, mode_cmd)


T_squat_start = 102;
T_climb_start = 130;

if (mode_cmd == 1) || (t < T_squat_start); q = 0; return; end

if t < T_climb_start
    tau = t - T_squat_start;
    q_stand = 0; q_squat = -deg2rad(70);
    T1 = 3; T2 = 15; T3 = 3;
    if tau < T1; u=tau/T1; q=(1-u)*q_stand+u*q_squat;
    elseif tau < T1+T2; q=q_squat;
    elseif tau < T1+T2+T3; u=(tau-(T1+T2))/T3; q=(1-u)*q_squat+u*q_stand;
    else; q=q_stand;
    end
    return;
end


tau = t - T_climb_start;

q_stand = deg2rad(0);
    q_lift  = deg2rad(-20);

   
    if tau < 10.0
        q = q_stand;
        
   
    elseif tau < 12.0
        dt = tau - 10.0;
        u = dt / 2.0;
        lift_scale = sin(u * pi);
        q = q_stand + lift_scale * (q_lift - q_stand);
        
    else
        q = q_stand;
    end
end

== matlab function DrivePurePursuitSquat/RR/Gait/MATLAB Function4 ==
  data: t input; w output
function w = wheel_speed(t)


Tsw  = 105;   
Tacc = 2;     
V    = 100;  
Tdec_start = 125;   
Tdec = 3;           

if t < Tsw
    w = 0;


elseif t < Tsw + Tacc
    u = (t - Tsw) / Tacc;
    w = u * V;

elseif t < Tdec_start
    w = V;

elseif t < Tdec_start + Tdec
    u = (t - Tdec_start) / Tdec; 
    w = V * (1 - u);

else
    w = 0;
end
end

== matlab function DrivePurePursuitSquat/FR/Wheel Lock/MATLAB Function5 ==
  settings: updateMethod=DISCRETE
  data: mode_cmd input; tau output; q input; dq input
function tau = WheelLockPD(mode_cmd, q, dq)
%#codegen
% mode_cmd: 0=Walk (lock wheel), 1=Wheeled (don't lock wheel)
% q, dq measurements from the wheel axle Revolute Joint
% Braking PD parameters (tunable)
Kp = 50.0;     % Braking stiffness, smaller to avoid being too rigid
Kd =  5.0;     % Damping
tau_lim = 150.0;  % Maximum braking torque for the wheel
% Lock only in walk mode
lock = (mode_cmd == 0);
persistent q_hold last_lock
if isempty(q_hold),    q_hold    = q;     end
if isempty(last_lock), last_lock = false; end
% The moment it switches from "unlocked" to "locked", remember the current angle
if (~last_lock) && lock
    q_hold = q;
end
last_lock = lock;
if lock
    % Lock wheel: treat q_hold as the target angle
    q_ref  = q_hold;
    dq_ref = 0.0;
    tau = Kp*(q_ref - q) + Kd*(dq_ref - dq);
else
    % Wheeled mode: do not apply brake
    tau = 0.0;
end
% Torque saturation
if tau >  tau_lim, tau =  tau_lim; end
if tau < -tau_lim, tau = -tau_lim; end
end

== matlab function DrivePurePursuitSquat/RL/MATLAB Function5 ==
  settings: updateMethod=DISCRETE
  data: mode_cmd input; tau output; q input; dq input
function tau = WheelLockPD(mode_cmd, q, dq)
%#codegen
% mode_cmd: 0=Walk (lock wheel), 1=Wheeled (don't lock wheel)
% q, dq measurements from the wheel axle Revolute Joint
% Braking PD parameters (tunable)
Kp = 50.0;     % Braking stiffness, smaller to avoid being too rigid
Kd =  5.0;     % Damping
tau_lim = 150.0;  % Maximum braking torque for the wheel
% Lock only in walk mode
lock = (mode_cmd == 0);
persistent q_hold last_lock
if isempty(q_hold),    q_hold    = q;     end
if isempty(last_lock), last_lock = false; end
% The moment it switches from "unlocked" to "locked", remember the current angle
if (~last_lock) && lock
    q_hold = q;
end
last_lock = lock;
if lock
    % Lock wheel: treat q_hold as the target angle
    q_ref  = q_hold;
    dq_ref = 0.0;
    tau = Kp*(q_ref - q) + Kd*(dq_ref - dq);
else
    % Wheeled mode: do not apply brake
    tau = 0.0;
end
% Torque saturation
if tau >  tau_lim, tau =  tau_lim; end
if tau < -tau_lim, tau = -tau_lim; end
end

== matlab function DrivePurePursuitSquat/RR/Gait/MATLAB Function5 ==
  settings: updateMethod=DISCRETE
  data: mode_cmd input; tau output; q input; dq input
function tau = WheelLockPD(mode_cmd, q, dq)
%#codegen
% mode_cmd: 0=Walk (lock wheel), 1=Wheeled (don't lock wheel)
% q, dq measurements from the wheel axle Revolute Joint
% Braking PD parameters (tunable)
Kp = 50.0;     % Braking stiffness, smaller to avoid being too rigid
Kd =  5.0;     % Damping
tau_lim = 150.0;  % Maximum braking torque for the wheel
% Lock only in walk mode
lock = (mode_cmd == 0);
persistent q_hold last_lock
if isempty(q_hold),    q_hold    = q;     end
if isempty(last_lock), last_lock = false; end
% The moment it switches from "unlocked" to "locked", remember the current angle
if (~last_lock) && lock
    q_hold = q;
end
last_lock = lock;
if lock
    % Lock wheel: treat q_hold as the target angle
    q_ref  = q_hold;
    dq_ref = 0.0;
    tau = Kp*(q_ref - q) + Kd*(dq_ref - dq);
else
    % Wheeled mode: do not apply brake
    tau = 0.0;
end
% Torque saturation
if tau >  tau_lim, tau =  tau_lim; end
if tau < -tau_lim, tau = -tau_lim; end
end

== matlab function DrivePurePursuitSquat/FL/MATLAB Function5 ==
  settings: updateMethod=DISCRETE
  data: mode_cmd input; tau output; q input; dq input
function tau = WheelLockPD(mode_cmd, q, dq)
%#codegen
% mode_cmd: 0=Walk (lock wheel), 1=Wheeled (don't lock wheel)
% q, dq measurements from the wheel axle Revolute Joint
% Braking PD parameters (tunable)
Kp = 50.0;     % Braking stiffness, smaller to avoid being too rigid
Kd =  5.0;     % Damping
tau_lim = 150.0;  % Maximum braking torque for the wheel
% Lock only in walk mode
lock = (mode_cmd == 0);
persistent q_hold last_lock
if isempty(q_hold),    q_hold    = q;     end
if isempty(last_lock), last_lock = false; end
% The moment it switches from "unlocked" to "locked", remember the current angle
if (~last_lock) && lock
    q_hold = q;
end
last_lock = lock;
if lock
    % Lock wheel: treat q_hold as the target angle
    q_ref  = q_hold;
    dq_ref = 0.0;
    tau = Kp*(q_ref - q) + Kd*(dq_ref - dq);
else
    % Wheeled mode: do not apply brake
    tau = 0.0;
end
% Torque saturation
if tau >  tau_lim, tau =  tau_lim; end
if tau < -tau_lim, tau = -tau_lim; end
end

== matlab function DrivePurePursuitSquat/RR/LockJointPD_h/MATLAB Function ==
  data: mode_cmd input; alpha input; tau output; q input; dq input; q_cmd input; is_locked output; q_ref output
function [tau, is_locked, q_ref] = LockJointPD(mode_cmd, alpha, q, dq, q_cmd)
%#codegen
% mode_cmd: 0=Walk(folloew q_cmd), 1=Wheel(lock the present angle )
% alpha   : [0,1] flatten faktor(TransferFcnoutput)，0=walk, 1=leg locked
% q,dq    : joint angle/angular velocity
% q_cmd   : walking/standing angle(rad)

Kp = 1200.0;   % start value
Kd =   20.0;
tau_lim = 300.0;

m = uint8(mode_cmd ~= 0);     % uint8(0/1)
a = double(alpha);

persistent q_hold last_mode
if isempty(q_hold),    q_hold    = q;        end   % double
if isempty(last_mode), last_mode = uint8(0); end   % uint8

% step: 0->1 
if (last_mode == uint8(0)) && (m ~= uint8(0))
    q_hold = q;
end
last_mode = m;

% reference angle
q_ref  = a*q_hold + (1-a)*q_cmd;
dq_ref = 0.0;

% PD
tau = Kp*(q_ref - q) + Kd*(dq_ref - dq);

% 
tau = max(min(tau, tau_lim), -tau_lim);

% 
is_locked = (a > 0.5);     % 
end

== matlab function DrivePurePursuitSquat/FR/LockJointPD_h/MATLAB Function ==
  data: mode_cmd input; alpha input; tau output; q input; dq input; q_cmd input; is_locked output; q_ref output
function [tau, is_locked, q_ref] = LockJointPD(mode_cmd, alpha, q, dq, q_cmd)
%#codegen
% mode_cmd: 0=Walk (track q_cmd), 1=Wheeled (lock current angle)
% alpha   : [0,1] smoothing factor (TransferFcn output), 0=fully walking, 1=fully locked
% q,dq    : joint angle/angular velocity
% q_cmd   : walk/stand target angle (radians)
Kp = 1200.0;   % Starting value, tune per joint
Kd =   20.0;
tau_lim = 300.0;
m = uint8(mode_cmd ~= 0);     % Standardize to uint8(0/1)
a = double(alpha);
persistent q_hold last_mode
if isempty(q_hold),    q_hold    = q;        end   % double
if isempty(last_mode), last_mode = uint8(0); end   % uint8
% Rising edge: 0->1, latch current angle
if (last_mode == uint8(0)) && (m ~= uint8(0))
    q_hold = q;
end
last_mode = m;
% Reference angle: interpolate between "hold angle" and "target angle"
q_ref  = a*q_hold + (1-a)*q_cmd;
dq_ref = 0.0;
% PD
tau = Kp*(q_ref - q) + Kd*(dq_ref - dq);
% Saturation
tau = max(min(tau, tau_lim), -tau_lim);
% Debug flag: is leg lock dominant
is_locked = (a > 0.5);     % Can also output m==1
end

== matlab function DrivePurePursuitSquat/FR/LockJointPD_k/MATLAB Function1 ==
  data: mode_cmd input; alpha input; tau output; q input; dq input; q_cmd input; is_locked output; q_ref output
function [tau, is_locked, q_ref] = LockJointPD(mode_cmd, alpha, q, dq, q_cmd)
%#codegen
% mode_cmd: 0=Walk (track q_cmd), 1=Wheeled (lock current angle)
% alpha   : [0,1] smoothing factor (TransferFcn output), 0=fully walking, 1=fully locked
% q,dq    : joint angle/angular velocity
% q_cmd   : walk/stand target angle (radians)
Kp = 1200.0;   % Starting value, tune per joint
Kd =   20.0;
tau_lim = 300.0;
m = uint8(mode_cmd ~= 0);     % Standardize to uint8(0/1)
a = double(alpha);
persistent q_hold last_mode
if isempty(q_hold),    q_hold    = q;        end   % double
if isempty(last_mode), last_mode = uint8(0); end   % uint8
% Rising edge: 0->1, latch current angle
if (last_mode == uint8(0)) && (m ~= uint8(0))
    q_hold = q;
end
last_mode = m;
% Reference angle: interpolate between "hold angle" and "target angle"
q_ref  = a*q_hold + (1-a)*q_cmd;
dq_ref = 0.0;
% PD
tau = Kp*(q_ref - q) + Kd*(dq_ref - dq);
% Saturation
tau = max(min(tau, tau_lim), -tau_lim);
% Debug flag: is leg lock dominant
is_locked = (a > 0.5);     % Can also output m==1
end

== matlab function DrivePurePursuitSquat/FL/MATLAB Function ==
  data: mode_cmd input; alpha input; tau output; q input; dq input; q_cmd input; is_locked output; q_ref output
function [tau, is_locked, q_ref] = LockJointPD(mode_cmd, alpha, q, dq, q_cmd)
%#codegen
% mode_cmd: 0=Walk (track q_cmd), 1=Wheeled (lock current angle)
% alpha   : [0,1] smoothing factor (TransferFcn output), 0=fully walking, 1=fully locked
% q,dq    : joint angle/angular velocity
% q_cmd   : walk/stand target angle (radians)
Kp = 1200.0;   % Starting value, tune per joint
Kd =   20.0;
tau_lim = 300.0;
m = uint8(mode_cmd ~= 0);     % Standardize to uint8(0/1)
a = double(alpha);
persistent q_hold last_mode
if isempty(q_hold),    q_hold    = q;        end   % double
if isempty(last_mode), last_mode = uint8(0); end   % uint8
% Rising edge: 0->1, latch current angle
if (last_mode == uint8(0)) && (m ~= uint8(0))
    q_hold = q;
end
last_mode = m;
% Reference angle: interpolate between "hold angle" and "target angle"
q_ref  = a*q_hold + (1-a)*q_cmd;
dq_ref = 0.0;
% PD
tau = Kp*(q_ref - q) + Kd*(dq_ref - dq);
% Saturation
tau = max(min(tau, tau_lim), -tau_lim);
% Debug flag: is leg lock dominant
is_locked = (a > 0.5);     % Can also output m==1
end

== matlab function DrivePurePursuitSquat/FL/MATLAB Function1 ==
  data: mode_cmd input; alpha input; tau output; q input; dq input; q_cmd input; is_locked output; q_ref output
function [tau, is_locked, q_ref] = LockJointPD(mode_cmd, alpha, q, dq, q_cmd)
%#codegen
% mode_cmd: 0=Walk (track q_cmd), 1=Wheeled (lock current angle)
% alpha   : [0,1] smoothing factor (TransferFcn output), 0=fully walking, 1=fully locked
% q,dq    : joint angle/angular velocity
% q_cmd   : walk/stand target angle (radians)
Kp = 1200.0;   % Starting value, tune per joint
Kd =   20.0;
tau_lim = 300.0;
m = uint8(mode_cmd ~= 0);     % Standardize to uint8(0/1)
a = double(alpha);
persistent q_hold last_mode
if isempty(q_hold),    q_hold    = q;        end   % double
if isempty(last_mode), last_mode = uint8(0); end   % uint8
% Rising edge: 0->1, latch current angle
if (last_mode == uint8(0)) && (m ~= uint8(0))
    q_hold = q;
end
last_mode = m;
% Reference angle: interpolate between "hold angle" and "target angle"
q_ref  = a*q_hold + (1-a)*q_cmd;
dq_ref = 0.0;
% PD
tau = Kp*(q_ref - q) + Kd*(dq_ref - dq);
% Saturation
tau = max(min(tau, tau_lim), -tau_lim);
% Debug flag: is leg lock dominant
is_locked = (a > 0.5);     % Can also output m==1
end

== matlab function DrivePurePursuitSquat/RL/MATLAB Function ==
  data: mode_cmd input; alpha input; tau output; q input; dq input; q_cmd input; is_locked output; q_ref output
function [tau, is_locked, q_ref] = LockJointPD(mode_cmd, alpha, q, dq, q_cmd)
%#codegen
% mode_cmd: 0=Walk (track q_cmd), 1=Wheeled (lock current angle)
% alpha   : [0,1] smoothing factor (TransferFcn output), 0=fully walking, 1=fully locked
% q,dq    : joint angle/angular velocity
% q_cmd   : walk/stand target angle (radians)
Kp = 1200.0;   % Starting value, tune per joint
Kd =   20.0;
tau_lim = 300.0;
m = uint8(mode_cmd ~= 0);     % Standardize to uint8(0/1)
a = double(alpha);
persistent q_hold last_mode
if isempty(q_hold),    q_hold    = q;        end   % double
if isempty(last_mode), last_mode = uint8(0); end   % uint8
% Rising edge: 0->1, latch current angle
if (last_mode == uint8(0)) && (m ~= uint8(0))
    q_hold = q;
end
last_mode = m;
% Reference angle: interpolate between "hold angle" and "target angle"
q_ref  = a*q_hold + (1-a)*q_cmd;
dq_ref = 0.0;
% PD
tau = Kp*(q_ref - q) + Kd*(dq_ref - dq);
% Saturation
tau = max(min(tau, tau_lim), -tau_lim);
% Debug flag: is leg lock dominant
is_locked = (a > 0.5);     % Can also output m==1
end
